simulink subsystem "PieroAJModelZ"  (R2023b)
settings: Solver=VariableStepAuto  StartTime=0.0  StopTime=10.0  RelTol=1e-3
settings Model: Creator=jaime  LastModifiedBy=jaime

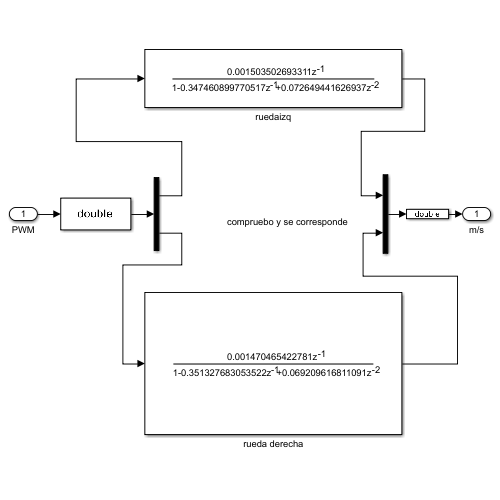
[thumbnail: Simulink's stored preview of the top-level diagram]
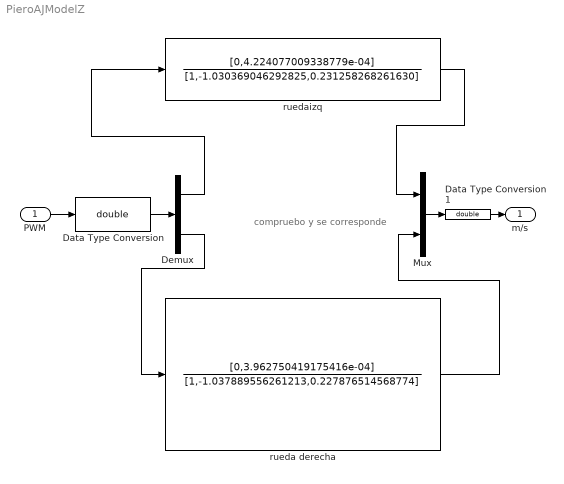
== system PieroAJModelZ ==
  note: compruebo y se corresponde
  PWM : Inport
  Data Type Conversion : DataTypeConversion  OutDataTypeStr=double  SaturateOnIntegerOverflow=off  RndMeth=Floor
  Data Type Conversion1 : DataTypeConversion  OutDataTypeStr=double  SaturateOnIntegerOverflow=off  RndMeth=Floor
  Demux : Demux  Outputs=2
  Mux : Mux  Inputs=2
  rueda derecha : DiscreteFilter  Numerator=[0,3.962750419175416e-04]  Denominator=[1,-1.037889556261213,0.227876514568774]
  ruedaizq : DiscreteFilter  Numerator=[0,4.224077009338779e-04]  Denominator=[1,-1.030369046292825,0.231258268261630]
  m/s : Outport
  wires:
  PWM/1 -> Data Type Conversion/1
  Data Type Conversion/1 -> Demux/1
  Mux/1 -> Data Type Conversion1/1
  Data Type Conversion1/1 -> m/s/1
  Demux/1 -> ruedaizq/1
  ruedaizq/1 -> Mux/1
  Demux/2 -> rueda derecha/1
  rueda derecha/1 -> Mux/2
